simulink subsystem "PieroModel"  (R2023b)
settings: Solver=VariableStepAuto  StartTime=0.0  StopTime=10.0  RelTol=1e-3
settings Model: Creator=manu_  LastModifiedBy=manu_

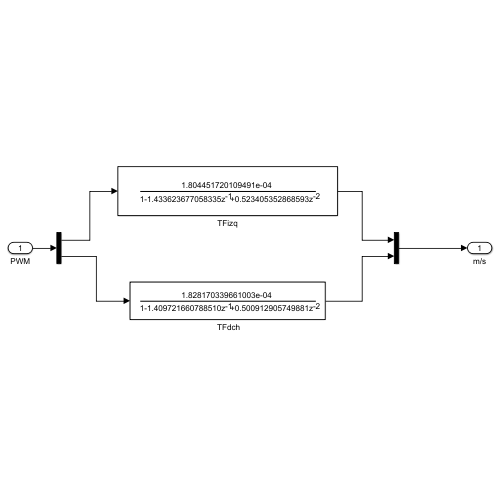
[thumbnail: Simulink's stored preview of the top-level diagram]
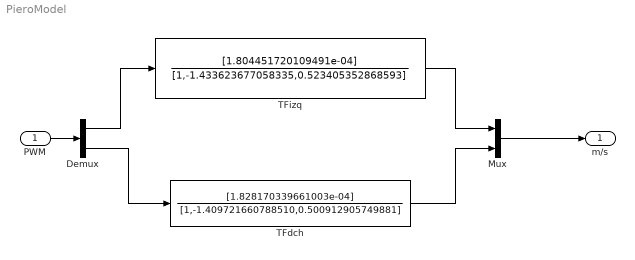
== system PieroModel ==
  PWM : Inport
  " TFdch" : DiscreteFilter  Numerator=[1.828170339661003e-04]  Denominator=[1,-1.409721660788510,0.500912905749881]
  Demux : Demux  Outputs=2
  Mux : Mux  Inputs=2
  TFizq : DiscreteFilter  Numerator=[1.804451720109491e-04]  Denominator=[1,-1.433623677058335,0.523405352868593]
  m/s : Outport
  wires:
  PWM/1 -> Demux/1
  Mux/1 -> m/s/1
  Demux/1 -> TFizq/1
  TFizq/1 -> Mux/1
  Demux/2 -> " TFdch"/1
  " TFdch"/1 -> Mux/2
